simulink model "deadbeat_running_control"  (R2016b)
settings: configuration reference "Configuration1khz" (kept outside this file)
undefined symbols (not defined in the file or in its folder): A_kalman_no_position, A_kalman_transverse, A_kalman_vertical, A_lpf_accelerometer, A_lpf_contact, A_lpf_imu, A_lpf_lateral_angle, B1_lpf_accelerometer, B1_lpf_contact, B1_lpf_imu, B1_lpf_lateral_angle, B2_lpf_accelerometer, B2_lpf_contact, B2_lpf_imu, B2_lpf_lateral_angle, B_dx_versus_x0, B_kalman_no_position, B_kalman_transverse, B_kalman_vertical, backwards_K_sag_of_t, backwards_P_sag_of_t, C_kalman_no_position, C_kalman_transverse, C_kalman_vertical, com_leg_motor, com_torso, contact_threshold, d_ankle_to_foot, d_vertical_com, desired_com_forward_velocity, desired_com_lateral_velocity, desired_standing_torso_pitch, desired_standing_torso_roll, desired_standing_z, desired_torso_pitch, desired_torso_roll, DiscIntNeverNeededParam, Discrete, enable_bouncing, fdesignblkfcn, flight_duration, forward_dx_of_dxstar, forward_x_of_dxstar, g, gcbh, HIP_MTR_MAX_CONT_TORQUE, HIP_MTR_MAX_TORQUE, i_leg_motor, i_robot, i_torso, initial_dx_estimate, initial_dx_takeoff_history, initial_dx_touchdown_history, initial_dy_estimate, initial_dy_takeoff_history, initial_dy_touchdown_history, initial_dz_estimate, initial_leg_selection, initial_target_dx_history, initial_target_dy_history ... (+80)
libraries: simulink x22, ctrlSharedLib x4, dsparch4 x2
(part 1 of 7)
settings Model: Creator=wmartin  LastModifiedBy=Will
settings ConfigSetRef: SourceLocation=Base Workspace

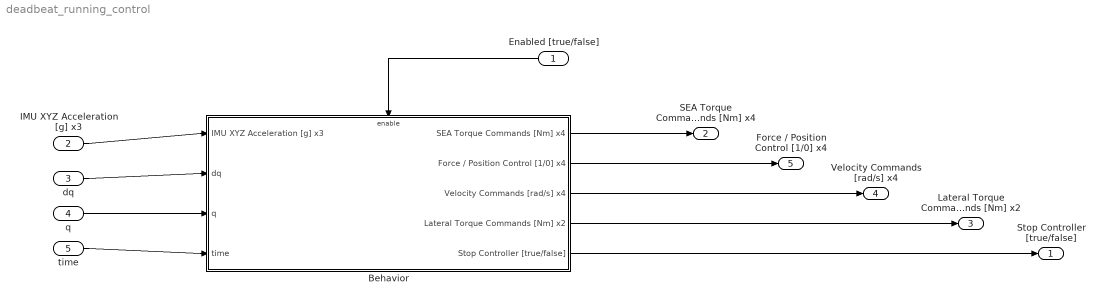
== system deadbeat_running_control ==
  Enabled [true/false] : Inport  OutDataTypeStr=boolean  PortDimensions=1  SampleTime=sample_time  Interpolate=off
  IMU XYZ Acceleration [g] x3 : Inport  Port=2  OutDataTypeStr=double  PortDimensions=3  SampleTime=[0.001,0]  Interpolate=off
  dq : Inport  Port=3  OutDataTypeStr=double  PortDimensions=13  SampleTime=[0.001,0]  Interpolate=off
  q : Inport  Port=4  OutDataTypeStr=double  PortDimensions=13  SampleTime=[0.001,0]  Interpolate=off
  time : Inport  Port=5  OutDataTypeStr=double  PortDimensions=1  SampleTime=sample_time  Interpolate=off
  Behavior : Subsystem
  Stop Controller [true/false] : Outport  OutDataTypeStr=boolean  PortDimensions=1  SampleTime=[0.001,0]  OutputWhenDisabled=reset  InitialOutput=[0 0 0 0 0 0]
  SEA Torque Commands [Nm] x4 : Outport  Port=2  OutDataTypeStr=double  PortDimensions=4  SampleTime=[0.001,0]  OutputWhenDisabled=reset  InitialOutput=[0 0 0 0 0 0]
  Lateral Torque Commands [Nm] x2 : Outport  Port=3  OutDataTypeStr=double  PortDimensions=2  SampleTime=[0.001,0]  OutputWhenDisabled=reset  InitialOutput=[0 0 0 0 0 0]
  Velocity Commands [rad/s] x4 : Outport  Port=4  OutDataTypeStr=double  PortDimensions=4  SampleTime=[0.001,0]  OutputWhenDisabled=reset  InitialOutput=[0 0 0 0 0 0]
  Force / Position Control [1/0] x4 : Outport  Port=5  OutDataTypeStr=boolean  PortDimensions=4  SampleTime=[0.001,0]  OutputWhenDisabled=reset  InitialOutput=[0 0 0 0 0 0]
  wires:
  IMU XYZ Acceleration [g] x3/1 -> Behavior/1(IMU XYZ Acceleration [g] x3)
  dq/1 -> Behavior/2(dq)
  q/1 -> Behavior/3(q)
  Behavior/1(SEA Torque Commands [Nm] x4) -> SEA Torque Commands [Nm] x4/1
  Behavior/2(Force / Position Control [1/0] x4) -> Force / Position Control [1/0] x4/1
  Behavior/3(Velocity Commands [rad/s] x4) -> Velocity Commands [rad/s] x4/1
  Behavior/4(Lateral Torque Commands [Nm] x2) -> Lateral Torque Commands [Nm] x2/1
  time/1 -> Behavior/4(time)
  Enabled [true/false]/1 -> Behavior/Enable
  Behavior/5(Stop Controller [true/false]) -> Stop Controller [true/false]/1

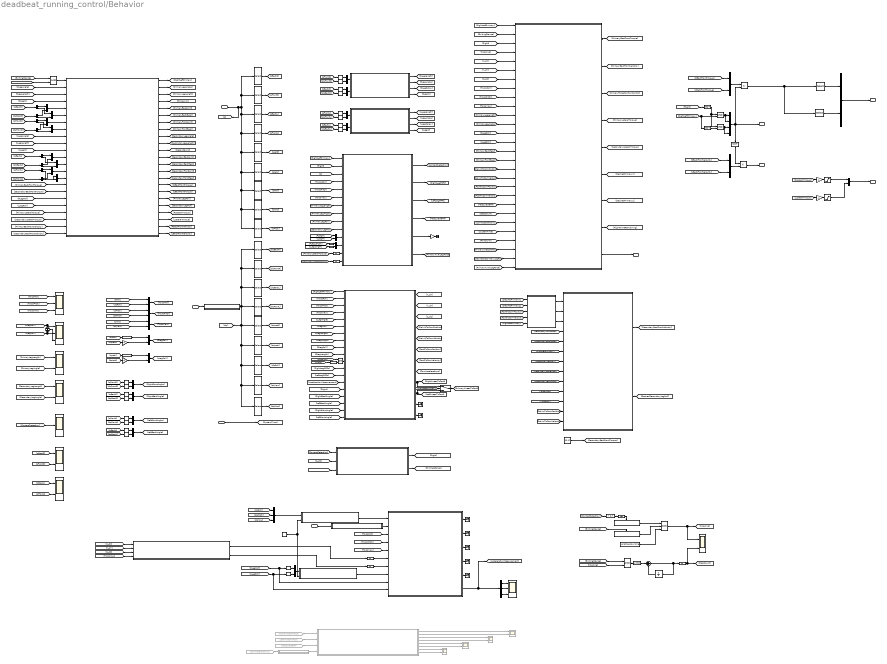
== system deadbeat_running_control/Behavior ==
  note: Signal Routing
  note: Begin Control
  note: Position & Velocity Estimation
  note: Force Estimation
  note: Leg/Spring Measurements
  note: Torque Commands
  note: Secondary Leg Behavior
  note: Primary Leg + Lateral Behavior
  note: Inputs
  note: q Order:
      |
      | backJointR
      | backGearR
      | frontJointR
      | frontGearR
      |
      | backJointL
      | backGearL
      | frontJointL
      | frontGearL
      |
      | latR
      | latL
      |
      | torsoRoll
      | torsoYaw
      | torsoPitch
  note: Angle Conversions
  note: Contact Estimation
  note: Logging
  note: Acceleration Measurement
  note: Knee Torque Estimation
  IMU XYZ Acceleration [g] x3 : Inport  OutDataTypeStr=double  PortDimensions=3  SampleTime=[0.001,0]
  dq : Inport  Port=2  OutDataTypeStr=double  PortDimensions=13  SampleTime=[0.001,0]
  q : Inport  Port=3  OutDataTypeStr=double  PortDimensions=13  SampleTime=[0.001,0]
  time : Inport  Port=4  OutDataTypeStr=double  PortDimensions=1  SampleTime=[0.001,0]
  Enable : EnablePort  PropagateVarSize=During execution  ShowOutputPort=on
  At Least One Stance Detected : Subsystem
  Atrias Swing control : Subsystem
  COM Acceleration Measurement : Scope  NumInputPorts=3
  Compare To Constant : simulink/Logic and Bit Operations/Compare To Constant  relop=>  const=0.7  OutDataTypeStr=boolean
  Compute Body Frame Accelerations : Subsystem
  Compute COM Translational Acceleration (IMU uses non-rotating measurement frame) : MATLAB Function  TreatAsAtomicUnit=on
  Compute Forces1 : Subsystem  Commented=on
  Compute World Frame COM Coordinates from Yawed Frame : MATLAB Function  TreatAsAtomicUnit=on
  Constant : Constant  Value=[0 0]
  Constant1 : Constant  Value=enable_bouncing
  Contact : Scope
  Contact State Machine : Subsystem
  Data Type Conversion : DataTypeConversion  OutDataTypeStr=uint32
  Demux : Demux  Outputs=3
  Demux{3..10} (8 alike) : Demux  Outputs=2
  Desired Secondary Swing Targets : Subsystem
  Estimate Angular Accelerations2 : Subsystem
  Estimate Angular Accelerations3 : Subsystem
  Exited Stance : Subsystem
  Filter Velocities : Subsystem
  Force Estimation : Subsystem
  From40 : From  Commented=on  GotoTag=RightKneesToFoot
  From56 : From  Commented=on  GotoTag=LeftKneesToFoot
  From57 : From  Commented=on  GotoTag=MeasuredGRF
  From76 : From  Commented=on  GotoTag=ComAccelerations
  Gain{1..2,12..13} (4 alike) : Gain  Gain=-1
  Hopping / Steps : Scope  NumInputPorts=2
  Knee Torques : MATLAB Function  Commented=on  TreatAsAtomicUnit=on
  L Knee Torques from Accelerometer : Scope  Commented=on  NumInputPorts=2
  L Knee Torques from Forward Dynamics : Scope  Commented=on  NumInputPorts=2
  L Leg Calculator : Subsystem
  Left Lateral Torque Saturation : Saturate  UpperLimit=max_torque_lateral  LowerLimit=-max_torque_lateral
      settings: AttributesFormatString=Top: %<UpperLimit>\nBottom: %<LowerLimit>
  Left Leg Fourbar Positions : Scope  NumInputPorts=2
  Logical Operator : Logic  IconShape=distinctive  AllPortsSameDT=off  OutDataTypeStr=boolean
  Logical Operator1 : Logic  AllPortsSameDT=off  OutDataTypeStr=boolean
  Logical Operator2 : Logic  Operator=OR  AllPortsSameDT=off  OutDataTypeStr=boolean
  Logical Operator3 : Logic  Inputs=3  AllPortsSameDT=off  OutDataTypeStr=boolean
  Logical Operator{4,6,8..9} (4 alike) : Logic  Operator=NOT  AllPortsSameDT=off  OutDataTypeStr=boolean
  Logical Operator5 : Logic  AllPortsSameDT=off  OutDataTypeStr=boolean
  Logical Operator7 : Logic  AllPortsSameDT=off  OutDataTypeStr=boolean
  Mux{,1..2,4..27,30} (28 alike) : Mux  Inputs=2
  Mux28 : Mux  Inputs=3
  Mux3 : Mux
  Primary Leg Length / Angle : Scope  NumInputPorts=2
  Primary Secondary Leg Swap : Subsystem
  Primary and Lateral Behavior : Subsystem
  Product : Product
  Product1 : Product
  R Knee Torques from Accelerometer : Scope  Commented=on  NumInputPorts=2
  R Knee Torques from Forward Dynamics : Scope  Commented=on  NumInputPorts=2
  R Leg Calculator : Subsystem
  Right Lateral Torque Saturation : Saturate  UpperLimit=max_torque_lateral  LowerLimit=-max_torque_lateral
      settings: AttributesFormatString=Top: %<UpperLimit>\nBottom: %<LowerLimit>
  Right Left Symmetry Leg Roll : Scope  NumInputPorts=3
  Right Leg Fourbar Positions : Scope  NumInputPorts=2
  Roll Pitch Yaw : Scope  NumInputPorts=3
  Secondary Leg Length / Angle : Scope  NumInputPorts=2
  Selector : Selector  InputPortWidth=4  IndexOptions=Index vector (dialog)  Indices=[1 2]  OutputSizes=1
  Selector1 : Selector  InputPortWidth=13  IndexOptions=Index vector (dialog)  Indices=[10]  OutputSizes=1
  Selector10 : Selector  InputPortWidth=13  IndexOptions=Index vector (dialog)  Indices=[7 8]  OutputSizes=1
  Selector11 : Selector  InputPortWidth=13  IndexOptions=Index vector (dialog)  Indices=[9]  OutputSizes=1
  Selector12 : Selector  InputPortWidth=13  IndexOptions=Index vector (dialog)  Indices=[1 2]  OutputSizes=1
  Selector13 : Selector  InputPortWidth=13  IndexOptions=Index vector (dialog)  Indices=[3 4]  OutputSizes=1
  Selector{14..17,19,24..27,29..37} (18 alike) : Selector  InputPortWidth=2  IndexOptions=Index vector (dialog)  Indices=[1]  OutputSizes=1
  Selector18 : Selector  InputPortWidth=13  IndexOptions=Index vector (dialog)  Indices=[13]  OutputSizes=1
  Selector2 : Selector  InputPortWidth=13  IndexOptions=Index vector (dialog)  Indices=[5 6]  OutputSizes=1
  Selector20 : Selector  InputPortWidth=13  IndexOptions=Index vector (dialog)  Indices=[13]  OutputSizes=1
  Selector21 : Selector  InputPortWidth=13  IndexOptions=Index vector (dialog)  Indices=[11]  OutputSizes=1
  Selector22 : Selector  InputPortWidth=13  IndexOptions=Index vector (dialog)  Indices=[12]  OutputSizes=1
  Selector23 : Selector  InputPortWidth=13  IndexOptions=Index vector (dialog)  Indices=[11]  OutputSizes=1
  Selector28 : Selector  InputPortWidth=13  IndexOptions=Index vector (dialog)  Indices=[12]  OutputSizes=1
  Selector3 : Selector  InputPortWidth=4  IndexOptions=Index vector (dialog)  Indices=[3 4]  OutputSizes=1
  Selector4 : Selector  InputPortWidth=13  IndexOptions=Index vector (dialog)  Indices=[7 8]  OutputSizes=1
  Selector41 : Selector  InputPortWidth=2  IndexOptions=Index vector (dialog)  Indices=[2]  OutputSizes=1
  Selector42 : Selector  InputPortWidth=2  IndexOptions=Index vector (dialog)  Indices=[2]  OutputSizes=1
  Selector5 : Selector  InputPortWidth=13  IndexOptions=Index vector (dialog)  Indices=[9]  OutputSizes=1
  Selector6 : Selector  InputPortWidth=13  IndexOptions=Index vector (dialog)  Indices=[1 2]  OutputSizes=1
  Selector7 : Selector  InputPortWidth=13  IndexOptions=Index vector (dialog)  Indices=[3 4]  OutputSizes=1
  Selector8 : Selector  InputPortWidth=13  IndexOptions=Index vector (dialog)  Indices=[10]  OutputSizes=1
  Selector9 : Selector  InputPortWidth=13  IndexOptions=Index vector (dialog)  Indices=[5 6]  OutputSizes=1
  State Estimation : Subsystem
  Sum1 : Sum  Inputs=|++  OutMin=0
  Sum3 : Sum  Inputs=-|+
  Switch : Switch  Criteria=u2 ~= 0
  Terminator{,1..7} (8 alike) : Terminator
  Unit Delay : UnitDelay  SampleTime=-1
  Unit Delay{1..6} (6 alike) : UnitDelay  SampleTime=sample_time
  lateral_coordinates : Fcn  Expr=pi/2-u
  lateral_coordinates1 : Fcn  Expr=pi/2-u
  torso_roll_acceleration : Gain
  SEA Torque Commands [Nm] x4 : Outport  OutDataTypeStr=double  PortDimensions=4  SampleTime=[0.001,0]  OutputWhenDisabled=reset  InitialOutput=[0 0 0 0]
  Force / Position Control [1/0] x4 : Outport  Port=2  OutDataTypeStr=boolean  PortDimensions=4  SampleTime=[0.001,0]  OutputWhenDisabled=reset  InitialOutput=[0 0 0 0]
  Velocity Commands [rad/s] x4 : Outport  Port=3  OutDataTypeStr=double  PortDimensions=4  SampleTime=[0.001,0]  OutputWhenDisabled=reset  InitialOutput=[0 0 0 0]
  Lateral Torque Commands [Nm] x2 : Outport  Port=4  OutDataTypeStr=double  PortDimensions=2  SampleTime=[0.001,0]  OutputWhenDisabled=reset  InitialOutput=[0 0]
  Stop Controller [true/false] : Outport  Port=5  OutDataTypeStr=boolean  PortDimensions=1  SampleTime=[0.001,0]  OutputWhenDisabled=reset  InitialOutput=0
  wires:
  [SecondaryLateralTorque] -> Unit Delay4/1
  Unit Delay3/1 -> Force Estimation/13(Primary Lateral Torque [Nm])
  Gain1/1 -> Left Lateral Torque Saturation/1
  [RLegLength] -> Selector19/1
  [RLegW] -> Mux19/1
  [PrimaryLateralTorque] -> Unit Delay3/1
  [PrimaryLateralTorque] -> Primary Secondary Leg Swap/20(Primary Lateral Torque [Nm])
  [SecondaryLegRoll] -> Force Estimation/10(Secondary Leg Roll [rad rad/s])
  Mux20/1 -> Force Estimation/12(Leg Length Right/Left [m m])
  Gain2/1 -> Right Lateral Torque Saturation/1
  [LLegRoll] -> Primary and Lateral Behavior/14(Left Leg Roll [rad rad/s])
  Selector29/1 -> Mux20/2
  Primary Secondary Leg Swap/20(Right Lateral Torque [Nm]) -> [RLateralTorque]
  Force Estimation/5(Torso Roll Acceleration [rad/s^2]) -> torso_roll_acceleration/1
  Primary and Lateral Behavior/4(Primary Lateral Torque [Nm]) -> [PrimaryLateralTorque]
  [SecondaryLateralTorque] -> Primary Secondary Leg Swap/21(Secondary Lateral Torque [Nm])
  Mux19/1 -> Force Estimation/11(Leg Width Right/Left [m m])
  Primary Secondary Leg Swap/21(Left Lateral Torque [Nm]) -> [LLateralTorque]
  torso_roll_acceleration/1 -> Terminator6/1
  Unit Delay4/1 -> Force Estimation/14(Secondary Lateral Torque [Nm])
  [Y_dY] -> Primary and Lateral Behavior/6("[y,  dy] [m, m/s]")
  [LLegLength] -> Selector29/1
  [StepCount] -> Primary and Lateral Behavior/22(Steps Taken)
  Logical Operator3/1 -> [hopping], Hopping / Steps/1
  [TorsoYaw] -> Primary and Lateral Behavior/10(Torso Yaw [rad rad/s])
  [RLegRoll] -> Primary and Lateral Behavior/13(Right Leg Roll [rad rad/s])
  [MeasuredGRF] -> Primary and Lateral Behavior/21(Measured GRF [N N N])
  [TorsoRoll] -> Primary and Lateral Behavior/8(Torso Roll [rad rad/s])
  [Z_dZ] -> Primary and Lateral Behavior/7("[z, dz] [m, m/s]")
  Selector19/1 -> Mux20/1
  Primary and Lateral Behavior/5(Secondary Lateral Torque [Nm]) -> [SecondaryLateralTorque]
  [LLegW] -> Mux19/2
  [RLegRoll] -> Right Left Symmetry Leg Roll/1, Sum3/1
  Mux23/1 -> [TorsoRoll]
  Mux7/1 -> [TorsoPitch]
  Contact State Machine/2(Exiting Stance [1/0]) -> [ExitingStance]
  [ContactDetection] -> Contact State Machine/1(Contact Factor [body weight])
  [PrimaryLegAngle] -> Primary and Lateral Behavior/12(Leg Angle [rad rad/s])
  [Z_dZ] -> Contact State Machine/2("[Z dZ] [m m/s]")
  [FootToComPosition] -> Primary and Lateral Behavior/19(Foot to COM Position [m m m])
  [PrimaryLegLength] -> Primary and Lateral Behavior/11(Leg Length [m m/s])
  [PrimaryFrontGear] -> Primary and Lateral Behavior/16(Primary Front Gear [rad rad/s])
  [hopping] -> Primary and Lateral Behavior/4(Hopping [1/0])
  [FootToComVelocity] -> Primary and Lateral Behavior/20(Foot to COM Velocity [m m m])
  [TorsoPitch] -> Roll Pitch Yaw/2
  [LLegRoll] -> Right Left Symmetry Leg Roll/2, Sum3/2
  [flight] -> Primary and Lateral Behavior/3(Flight [1/0])
  [TorsoPitch] -> Primary and Lateral Behavior/9(Torso Pitch [rad rad/s])
  Sum3/1 -> Right Left Symmetry Leg Roll/3
  [PrimaryLegLength] -> Primary Leg Length / Angle/1
  [PelvisToComPosition] -> Primary and Lateral Behavior/17(Pelvis to COM Position [m m m])
  [PrimaryLegAngle] -> Primary Leg Length / Angle/2
  [SecondaryLegLength] -> Secondary Leg Length / Angle/1
  [SecondaryLegAngle] -> Secondary Leg Length / Angle/2
  [ContactDetection] -> Contact/1
  Contact State Machine/1(flight [1/0]) -> [flight]
  [RightLeftPrimary] -> Primary and Lateral Behavior/1(Right/Left [1/0])
  [X_dX] -> Primary and Lateral Behavior/5("[x, dx] [m, m/s]")
  [ExitingStance] -> Primary and Lateral Behavior/2(Exiting Stance [1/0])
  [TorsoRoll] -> Roll Pitch Yaw/1
  Mux21/1 -> [TorsoYaw]
  [PelvisToComVelocity] -> Primary and Lateral Behavior/18(Pelvis to COM Velocity [m m m])
  [PrimaryBackGear] -> Primary and Lateral Behavior/15(Primary Back Gear [rad rad/s])
  [TorsoYaw] -> Roll Pitch Yaw/3
  [dqLatL] -> Gain13/1
  Selector21/1 -> [dqRoll]
  Selector9/1 -> [dqBackL]
  [qYaw] -> Mux21/1
  time/1 -> [SystemTime]
  [dqLatR] -> Gain12/1
  lateral_coordinates/1 -> Mux22/1
  [ComAccelerations] -> Primary and Lateral Behavior/23(COM XYZ Acceleration [m/s^2] x3)
  [qBackL] -> Left Leg Fourbar Positions/1
  Gain12/1 -> Mux22/2
  [dqPitch] -> Mux7/2
  Selector20/1 -> [dqPitch]
  [qRoll] -> Mux23/1
  [qPitch] -> Mux7/1
  lateral_coordinates1/1 -> Mux24/1
  Selector10/1 -> [dqFrontL]
  [qBackR] -> Right Leg Fourbar Positions/1
  [qLatL] -> lateral_coordinates1/1
  Mux22/1 -> [RLegRoll]
  Gain13/1 -> Mux24/2
  Selector13/1 -> [dqFrontR]
  Selector11/1 -> [dqLatR]
  Mux24/1 -> [LLegRoll]
  [dqRoll] -> Mux23/2
  Selector8/1 -> [dqLatL]
  [dqYaw] -> Mux21/2
  [qLatR] -> lateral_coordinates/1
  [qFrontR] -> Right Leg Fourbar Positions/2
  Selector12/1 -> [dqBackR]
  Selector22/1 -> [dqYaw]
  [qFrontL] -> Left Leg Fourbar Positions/2
  Atrias Swing control/2(Desired Swing Beta [rad rad/s rad/s^2]) -> [DesiredSecondaryLegRoll]
  [DesiredPrimaryX] -> Desired Secondary Swing Targets/1(Desired Primary X)
  Atrias Swing control/1(Secondary Back/Front Motor Velocity [rad/s rad/s]) -> [SecondaryBackFrontVelocity]
  Desired Secondary Swing Targets/2(Desired Y) -> Atrias Swing control/2(Y Desired [m m/s m/s^2])
  State Estimation/12(Foot to COM Velocity Global [m/s m/s m/s]) -> Terminator1/1
  Primary and Lateral Behavior/6("Desired Primary X [m, m/s, m/s^2]") -> [DesiredPrimaryX]
  Desired Secondary Swing Targets/3(Desired Z) -> Atrias Swing control/3(Z Desired [m m/s m/s^2])
  Desired Secondary Swing Targets/1(Desired X) -> Atrias Swing control/1(X Desired [m m/s m/s^2])
  Primary and Lateral Behavior/7("Desired Primary Z [m, m/s, m/s^2]") -> [DesiredPrimaryZ]
  State Estimation/11(Foot to COM Position Global [m m m]) -> Terminator/1
  [DesiredPrimaryZ] -> Desired Secondary Swing Targets/2(Desired Primary Z)
  [FootToComPosition] -> Desired Secondary Swing Targets/3(Primary X,Y,Z)
  [PrimaryAxialLegForce] -> Primary and Lateral Behavior/28(Primary Axial Leg Force [N])
  Force Estimation/6(Primary Axial Leg Force) -> [PrimaryAxialLegForce]
  [FootToComVelocity] -> Desired Secondary Swing Targets/4(Primary dX,dY,dZ)
  [DesiredSecondaryLegRoll] -> Primary and Lateral Behavior/27(Desired Secondary Leg Roll [rad rad/s rad/s^2])
  [RightLeftPrimary] -> Desired Secondary Swing Targets/5(Right / Left)
  [PelvisToComVelocity] -> Atrias Swing control/13(Pelvis to COM Velocity [m/s m/s m/s])
  [PelvisToComPosition] -> Atrias Swing control/12(Pelvis to COM Position [m m m])
  Compute World Frame COM Coordinates from Yawed Frame/2(com_velocity_world) -> Unit Delay6/1
  Selector42/1 -> Mux30/2
  [LLegRoll] -> Selector42/1, Compute COM Translational Acceleration (IMU uses non-rotating measurement frame)/10(left_hip_roll)
  [TorsoYaw] -> Compute COM Translational Acceleration (IMU uses non-rotating measurement frame)/5(torso_yaw)
  [TorsoRoll] -> Atrias Swing control/11(Torso Roll [rad rad/s])
  [SecondaryLegLength] -> Atrias Swing control/8(Secondary Leg Length [m m/s])
  [SecondaryLegAngle] -> Atrias Swing control/9(Secondary Leg Angle [rad rad/s])
  Compute World Frame COM Coordinates from Yawed Frame/1(com_position_world) -> Unit Delay5/1
  Unit Delay6/1 -> Compute COM Translational Acceleration (IMU uses non-rotating measurement frame)/7(com_velocity_world)
  Unit Delay5/1 -> Compute COM Translational Acceleration (IMU uses non-rotating measurement frame)/6(com_position_world)
  [TorsoPitch] -> Atrias Swing control/10(Torso Pitch [rad rad/s])
  [RightLeftPrimary] -> Atrias Swing control/6(Right or Left Stance [1 or 0])
  [TorsoYaw] -> Compute World Frame COM Coordinates from Yawed Frame/4(torso_yaw)
  [X_dX] -> Compute World Frame COM Coordinates from Yawed Frame/1(X_dX)
  Estimate Angular Accelerations3/1(Angular Accelerations [rad/s^2] x2) -> Compute COM Translational Acceleration (IMU uses non-rotating measurement frame)/8(hip_roll_accelerations)
  Mux30/1 -> Estimate Angular Accelerations3/1(Angular Velocities [rad/s] x2)
  [SecondaryLegRoll] -> Atrias Swing control/7(Secondary Leg Roll [rad rad/s])
  [Y_dY] -> Compute World Frame COM Coordinates from Yawed Frame/2(Y_dY)
  Selector41/1 -> Mux30/1
  Estimate Angular Accelerations2/1(Angular Accelerations [rad/s^2] x3) -> Compute COM Translational Acceleration (IMU uses non-rotating measurement frame)/1(torso_angular_accelerations)
  IMU XYZ Acceleration [g] x3/1 -> Compute Body Frame Accelerations/1(accelerometer [g] x3)
  [RLegRoll] -> Selector41/1, Compute COM Translational Acceleration (IMU uses non-rotating measurement frame)/9(right_hip_roll)
  Mux28/1 -> Estimate Angular Accelerations2/1(Angular Velocities [rad/s] x3)
  [dqYaw] -> Mux28/3
  [Z_dZ] -> Compute World Frame COM Coordinates from Yawed Frame/3(Z_dZ)
  Enable/1 -> Estimate Angular Accelerations2/2(Enabled), Estimate Angular Accelerations3/2(Enabled)
  [SecondaryBackGear] -> Atrias Swing control/5(Secondary Back Gear [rad rad/s])
  [dqPitch] -> Mux28/2
  [dqRoll] -> Mux28/1
  [SecondaryFrontGear] -> Atrias Swing control/4(Secondary Front Gear [rad rad/s])
  Compute COM Translational Acceleration (IMU uses non-rotating measurement frame)/6(com_acceleration_yawed) -> Demux/1, [AccelerationMeasurement]
  Logical Operator2/1 -> State Estimation/11(Enable Kalman Filtering [1/0])
  [RightLegGRFs] -> State Estimation/12(Right GRF [X Y Z] [N N N])
  [RLegAngle] -> State Estimation/8(Right Leg Sagittal Angle [rad rad/s])
  Switch/1 -> [PrimaryKneesToFoot]
  State Estimation/8(COM Acceleration [m/s^2] x3) -> [ComAccelerations]
  State Estimation/1("Horizontal COM [m, m/s]") -> [X_dX]
  [RLegRoll] -> State Estimation/9(Right Leg Roll [rad rad/s])
  [AccelerationMeasurement] -> State Estimation/14(" Acceleration Measurement [m/s^2] x3")
  [LeftFrontAngle] -> State Estimation/19(Left Front [rad rad/s])
  [RightBackAngle] -> State Estimation/16(Right Back [rad rad/s])
  Demux/3 -> COM Acceleration Measurement/3
  [RightLeftPrimary] -> Switch/2
  [TorsoRoll] -> Compute COM Translational Acceleration (IMU uses non-rotating measurement frame)/3(torso_roll)
  [RLegLength] -> State Estimation/10(Right Leg Length [m m/s])
  [RightFrontAngle] -> State Estimation/18(Right Front [rad rad/s])
  [TorsoPitch] -> Compute COM Translational Acceleration (IMU uses non-rotating measurement frame)/4(torso_pitch)
  Demux/2 -> COM Acceleration Measurement/2
  [TorsoRoll] -> State Estimation/2(Torso Roll [rad rad/s])
  [TorsoPitch] -> State Estimation/3(Torso Pitch [rad rad/s])
  Demux/1 -> COM Acceleration Measurement/1
  [LLegRoll] -> State Estimation/6(Left Leg Roll [rad rad/s])
  [LLegLength] -> State Estimation/7(Left Leg Length [m m/s])
  [LLegAngle] -> State Estimation/5(Left Leg Sagittal Angle [rad rad/s])
  [RightLeftPrimary] -> State Estimation/1(Right or Left [1/0])
  State Estimation/9(Right Knees to Foot [m m m] x2) -> [RightKneesToFoot], Switch/1
  State Estimation/10(Left Knees to Foot [m m m] x2) -> Switch/3, [LeftKneesToFoot]
  [LeftBackAngle] -> State Estimation/17(Left Back [rad rad/s])
  State Estimation/3("Vertical COM [m, m/s]") -> [Z_dZ]
  Primary and Lateral Behavior/3(Primary Force or Position Control [1/0]) -> [PrimaryForcePositionControl]
  Logical Operator/1 -> Primary Secondary Leg Swap/1(Exiting Stance [1/0])
  [flight] -> Logical Operator4/1
  Primary and Lateral Behavior/1(Primary Back/Front SEA Torques [Nm] x2) -> [PrimaryBackFrontTorque]
  Sum1/1 -> Unit Delay2/1, Unit Delay/1
  Primary Secondary Leg Swap/16(R Back/Front SEA Torque [Nm Nm]) -> [RBackFrontTorque]
  State Estimation/4(Pelvis to COM Position [m m m]) -> [PelvisToComPosition]
  Logical Operator1/1 -> Data Type Conversion/1
  Primary Secondary Leg Swap/13(Secondary Back Gear [rad rad/s]) -> [SecondaryBackGear]
  [TorsoYaw] -> State Estimation/4(Torso Yaw [rad rad/s])
  [hopping] -> Logical Operator2/1
  [ExitingStance] -> Exited Stance/Enable
  [LeftLegGRFs] -> State Estimation/13(Left GRF [X Y Z] [N N N])
  State Estimation/5(Pelvis to COM Velocity [m/s m/s m/s]) -> [PelvisToComVelocity]
  [flight] -> State Estimation/15(Flight [1/0])
  State Estimation/7(Foot to COM Velocity [m/s m/s m/s]) -> [FootToComVelocity]
  Unit Delay/1 -> Sum1/2
  [RLateralTorque] -> Gain2/1
  Primary Secondary Leg Swap/17(L Back/Front SEA Torque [Nm Nm]) -> [LBackFrontTorque]
  State Estimation/2("Lateral COM [m, m/s]") -> [Y_dY]
  Logical Operator4/1 -> Logical Operator2/2
  Primary Secondary Leg Swap/11(Secondary Leg w [m]) -> [SecondaryW]
  Primary Secondary Leg Swap/15(Secondary Front Gear [rad rad/s]) -> [SecondaryFrontGear]
  State Estimation/6(Foot to COM Position [m m m]) -> [FootToComPosition]
  Primary Secondary Leg Swap/14(Secondary Front Joint [rad rad/s]) -> [SecondaryFrontJoint]
  Primary Secondary Leg Swap/1(Right/Left Primary [1/0]) -> [RightLeftPrimary]
  Data Type Conversion/1 -> Sum1/1
  Primary Secondary Leg Swap/12(Secondary Back Joint [rad rad/s]) -> [SecondaryBackJoint]
  Primary Secondary Leg Swap/8(Primary Front Gear [rad rad/s]) -> [PrimaryFrontGear]
  Primary Secondary Leg Swap/7(Primary Front Joint [rad rad/s]) -> [PrimaryFrontJoint]
  Primary Secondary Leg Swap/6(Primary Back Gear [rad rad/s]) -> [PrimaryBackGear]
  Mux15/1 -> Primary Secondary Leg Swap/15(L Front Gear [rad rad/s])
  Mux12/1 -> Primary Secondary Leg Swap/8(R Front Gear [rad rad/s])
  Mux11/1 -> Primary Secondary Leg Swap/7(R Front Joint [rad rad/s])
  Demux7/1 -> Mux14/1
  Mux10/1 -> Primary Secondary Leg Swap/6(R Back Gear [rad rad/s])
  Demux7/2 -> Mux15/1
  [SecondaryBackFrontTorque] -> Primary Secondary Leg Swap/17(Secondary Back/Front SEA Torque [Nm Nm])
  Mux14/1 -> Primary Secondary Leg Swap/14(L Front Joint [rad rad/s])
  Primary Secondary Leg Swap/5(Primary Back Joint [rad rad/s]) -> [PrimaryBackJoint]
  Demux10/2 -> Mux13/1
  Mux16/1 -> Primary Secondary Leg Swap/12(L Back Joint [rad rad/s])
  Demux6/2 -> Mux10/1
  Demux5/1 -> Mux9/2
  [qBackR] -> Demux6/1
  [dqBackL] -> Demux9/1
  [qBackL] -> Demux10/1
  Mux13/1 -> Primary Secondary Leg Swap/13(L Back Gear [rad rad/s])
  [dqFrontL] -> Demux8/1
  Demux8/2 -> Mux15/2
  Demux8/1 -> Mux14/2
  [dqBackR] -> Demux5/1
  Demux4/2 -> Mux12/2
  [qFrontL] -> Demux7/1
  Demux4/1 -> Mux11/2
  Demux10/1 -> Mux16/1
  Demux9/2 -> Mux13/2
  [PrimaryBackFrontTorque] -> Primary Secondary Leg Swap/16(Primary Back/Front SEA Torque [Nm Nm])
  Demux6/1 -> Mux9/1
  Demux5/2 -> Mux10/2
  Demux9/1 -> Mux16/2
  Demux3/2 -> Mux12/1
  Demux3/1 -> Mux11/1
  Selector27/1 -> Mux4/2
  Selector23/1 -> [qRoll]
  Mux9/1 -> Primary Secondary Leg Swap/5(R Back Joint [rad rad/s])
  [LLegLength] -> Primary Secondary Leg Swap/10(L Leg Length [m m/s])
  [dqFrontR] -> Demux4/1
  [qFrontR] -> Demux3/1
  [qBackL] -> Selector26/1
  Primary Secondary Leg Swap/2(Primary Leg Angle [rad rad/s]) -> [PrimaryLegAngle]
  [RLegLength] -> Primary Secondary Leg Swap/3(R Leg Length [m m/s])
  Selector25/1 -> Mux5/2
  Mux4/1 -> L Leg Calculator/2(Back [rad rad/s])
  [dqBackL] -> Selector27/1
  L Leg Calculator/4(w [m]) -> [LLegW]
  Mux5/1 -> L Leg Calculator/1(Front [rad rad/s])
  q/1 -> Selector6/1, Selector7/1, Selector2/1, Selector4/1, Selector5/1, Selector18/1, Selector28/1, Selector23/1, Selector1/1, [q]
  Selector24/1 -> Mux5/1
  [LLegAngle] -> Primary Secondary Leg Swap/9(L Leg Angle [rad rad/s])
  [LLegW] -> Primary Secondary Leg Swap/11(L Leg w [m])
  Primary Secondary Leg Swap/3(Primary Leg Length [m m/s]) -> [PrimaryLegLength]
  Primary Secondary Leg Swap/4(Primary Leg w [m]) -> [PrimaryW]
  Primary Secondary Leg Swap/10(Secondary Leg Length [rad rad/s]) -> [SecondaryLegLength]
  R Leg Calculator/4(w [m]) -> [RLegW]
  Selector26/1 -> Mux4/1
  L Leg Calculator/3(Leg Splay [rad rad/s]) -> [LLegSplay]
  L Leg Calculator/2(Leg Angle [rad rad/s]) -> [LLegAngle]
  L Leg Calculator/1("Leg Length [m m/s] ") -> [LLegLength]
  [qFrontL] -> Selector24/1
  Selector18/1 -> [qPitch]
  [dqFrontL] -> Selector25/1
  Primary Secondary Leg Swap/9(Secondary Leg Angle [rad rad/s]) -> [SecondaryLegAngle]
  [RLegW] -> Primary Secondary Leg Swap/4(R Leg w [m])
  [RLegAngle] -> Primary Secondary Leg Swap/2(R Leg Angle [rad rad/s])
  R Leg Calculator/3(Leg Splay [rad rad/s]) -> [RLegSplay]
  [dqBackR] -> Selector17/1
  Force Estimation/3(Left GRF [X Y Z] [N N N]) -> [LeftLegGRFs]
  Selector16/1 -> Mux1/1
  [LLateralTorque] -> Gain1/1
  Primary Secondary Leg Swap/19("Secondary Leg Roll [rad, rad/s]") -> [SecondaryLegRoll]
  Mux1/1 -> R Leg Calculator/2(Back [rad rad/s])
  Selector14/1 -> Mux2/1
  [qBackR] -> Selector16/1
  Selector2/1 -> [qBackL]
  Mux2/1 -> R Leg Calculator/1(Front [rad rad/s])
  Force Estimation/2(Right GRF [X Y Z] [N N N]) -> [RightLegGRFs]
  Selector4/1 -> [qFrontL]
  Selector5/1 -> [qLatR]
  Selector7/1 -> [qFrontR]
  Selector17/1 -> Mux1/2
  R Leg Calculator/2(Leg Angle [rad rad/s]) -> [RLegAngle]
  R Leg Calculator/1("Leg Length [m m/s] ") -> [RLegLength]
  Selector1/1 -> [qLatL]
  [dqFrontR] -> Selector15/1
  Selector6/1 -> [qBackR]
  [qFrontR] -> Selector14/1
  Force Estimation/1(Leg Plane Force for Contact Detection [body weight]) -> [ContactDetection]
  Force Estimation/4(GRF XYZ estimates [N N N]) -> [MeasuredGRF]
  [RLegRoll] -> Primary Secondary Leg Swap/18("Right Leg Roll [rad, rad/s]")
  Primary Secondary Leg Swap/18("Primary Leg Roll [rad, rad/s]") -> [PrimaryLegRoll]
  [LLegRoll] -> Primary Secondary Leg Swap/19("Left Leg Roll [rad, rad/s]")
  Unit Delay2/1 -> [StepCount], Hopping / Steps/2
  Selector28/1 -> [qYaw]
  Selector15/1 -> Mux2/2
  [PrimaryLegLength] -> Force Estimation/7(Primary Leg Length [m m/s])
  [PrimaryLegAngle] -> Force Estimation/8(Primary Leg Angle [rad rad/s])
  [PrimaryLegRoll] -> Force Estimation/9(Primary Leg Roll [rad rad/s])
  [ExitingStance] -> Logical Operator1/1
  [ExitingStance] -> Logical Operator/1
  [RightLeftPrimary] -> Force Estimation/1(Right/Left Primary)
  [flight] -> Force Estimation/2(Flight [1/0])
  [hopping] -> Logical Operator1/2
  [TorsoRoll] -> Force Estimation/4(Torso Roll [rad rad/s])
  [hopping] -> Logical Operator/2
  [TorsoYaw] -> Force Estimation/6(Torso Yaw [rad rad/s])
  [TorsoPitch] -> Force Estimation/5(Torso Pitch [rad rad/s])
  [q] -> Force Estimation/3(q)
  [RightLeftPrimary] -> Logical Operator5/2, Logical Operator8/1
  [RBackFrontVelocity] -> Mux6/1
  Unit Delay1/1 -> At Least One Stance Detected/Enable
  [LBackFrontVelocity] -> Mux6/2
  At Least One Stance Detected/1(Stance?) -> Logical Operator3/1
  [PrimaryBackFrontVelocity] -> Primary Secondary Leg Swap/22(Primary Front/Back Velocity [rad/s rad/s])
  [SecondaryBackFrontVelocity] -> Primary Secondary Leg Swap/23(Secondary Front/Back Velocity [rad/s rad/s])
  Primary Secondary Leg Swap/23(Left Front/Back Velocity [rad/s rad/s]) -> [LBackFrontVelocity]
  Selector3/1 -> Mux/2
  [SystemTime] -> Primary and Lateral Behavior/24(System Time [s])
  [PrimaryW] -> Primary and Lateral Behavior/25(Primary Leg Width [m])
  Exited Stance/1(Takeoff?) -> Logical Operator3/2
  [flight] -> Logical Operator6/1
  Compare To Constant/1 -> Unit Delay1/1
  Logical Operator8/1 -> Logical Operator7/2
  Logical Operator9/1 -> Product/1
  Mux/1 -> SEA Torque Commands [Nm] x4/1
  Product/1 -> Velocity Commands [rad/s] x4/1
  Primary and Lateral Behavior/2(Primary Back/Front Gear Velocities [rad/s] x2) -> [PrimaryBackFrontVelocity]
  [RBackFrontTorque] -> Mux8/1
  Mux6/1 -> Product/2
  [LBackFrontTorque] -> Mux8/2
  Product1/1 -> Selector/1, Selector3/1
  Primary Secondary Leg Swap/22(Right Front/Back Velocity [rad/s rad/s]) -> [RBackFrontVelocity]
  Selector/1 -> Mux/1
  Mux8/1 -> Product1/1
  Logical Operator7/1 -> Mux3/3, Mux3/4
  Constant/1 -> [SecondaryBackFrontTorque]
  Logical Operator5/1 -> Mux3/1, Mux3/2
  Logical Operator6/1 -> Logical Operator5/1, Logical Operator7/1
  Mux3/1 -> Force / Position Control [1/0] x4/1, Product1/2, Logical Operator9/1
  [ContactDetection] -> Compare To Constant/1
  [qFrontL] -> Selector34/1
  Knee Torques/6(left_back_knee_torques_from_fd) -> L Knee Torques from Forward Dynamics/2
  [dqFrontL] -> Selector35/1
  Selector34/1 -> Mux27/1
  Selector35/1 -> Mux27/2
  Knee Torques/2(right_back_knee_torques_from_fd) -> R Knee Torques from Forward Dynamics/2
  Compute Forces1/1(XYZ Force) -> Knee Torques/4(grf_from_accelerometer)
  From76/1 -> Compute Forces1/1(XYZ Acceleration)
  From40/1 -> Knee Torques/1(right_knees_to_foot)
  Knee Torques/1(right_front_knee_torques_from_fd) -> R Knee Torques from Forward Dynamics/1
  From57/1 -> Knee Torques/3(grf_from_seas)
  [dqBackR] -> Selector33/1
  [dqFrontR] -> Selector31/1
  Selector32/1 -> Mux17/1
  [qBackR] -> Selector32/1
  [dqBackL] -> Selector37/1
  Selector37/1 -> Mux26/2
  Selector31/1 -> Mux18/2
  [qBackL] -> Selector36/1
  Knee Torques/8(left_back_knee_torques_from_accelerometer) -> L Knee Torques from Accelerometer/2
  Selector36/1 -> Mux26/1
  [qFrontR] -> Selector30/1
  Knee Torques/4(right_back_knee_torques_from_accelerometer) -> R Knee Torques from Accelerometer/2
  Knee Torques/3(right_front_knee_torques_from_accelerometer) -> R Knee Torques from Accelerometer/1
  Selector30/1 -> Mux18/1
  Knee Torques/5(left_front_knee_torques_from_fd) -> L Knee Torques from Forward Dynamics/1
  Selector33/1 -> Mux17/2
  Knee Torques/7(left_front_knee_torques_from_accelerometer) -> L Knee Torques from Accelerometer/1
  From56/1 -> Knee Torques/2(left_knees_to_foot)
  [FlightTimeRemaining] -> Contact State Machine/3(Flight Time Remaining [s])
  Right Lateral Torque Saturation/1 -> Mux25/1
  Mux26/1 -> [LeftBackAngle]
  Mux17/1 -> [RightBackAngle]
  Mux18/1 -> [RightFrontAngle]
  dq/1 -> Filter Velocities/1(raw dq)
  Mux25/1 -> Lateral Torque Commands [Nm] x2/1
  [PrimaryKneesToFoot] -> Primary and Lateral Behavior/26(Primary Knees to Foot [m] x6)
  Mux27/1 -> [LeftFrontAngle]
  Compute Body Frame Accelerations/1(accelerations [m/s^2] x3) -> Compute COM Translational Acceleration (IMU uses non-rotating measurement frame)/2(imu_translational_accelerations_body)
  Filter Velocities/1(filtered dq) -> Selector9/1, Selector13/1, Selector12/1, Selector8/1, Selector22/1, Selector20/1, Selector21/1, Selector11/1, [dq], Selector10/1
  Left Lateral Torque Saturation/1 -> Mux25/2
  Compute COM Translational Acceleration (IMU uses non-rotating measurement frame)/2(torso_com_acceleration_world) -> Terminator3/1
  Compute COM Translational Acceleration (IMU uses non-rotating measurement frame)/3(pelvis_acceleration_world) -> Terminator4/1
  Compute COM Translational Acceleration (IMU uses non-rotating measurement frame)/4(right_hip_acceleration_world) -> Terminator5/1
  Compute COM Translational Acceleration (IMU uses non-rotating measurement frame)/1(com_acceleration_world) -> Terminator2/1
  Compute COM Translational Acceleration (IMU uses non-rotating measurement frame)/5(left_hip_acceleration_world) -> Terminator7/1
  Constant1/1 -> Logical Operator3/3
  Primary and Lateral Behavior/8(Flight Time Remaining [s]) -> [FlightTimeRemaining]
  Primary and Lateral Behavior/9(Stop Controller [true/false]) -> Stop Controller [true/false]/1

== system deadbeat_running_control/Behavior/At Least One Stance Detected ==
  Enable : EnablePort  StatesWhenEnabling=reset
  Constant : Constant
  Stance? : Outport  InitialOutput=[0]
  wires:
  Constant/1 -> Stance?/1

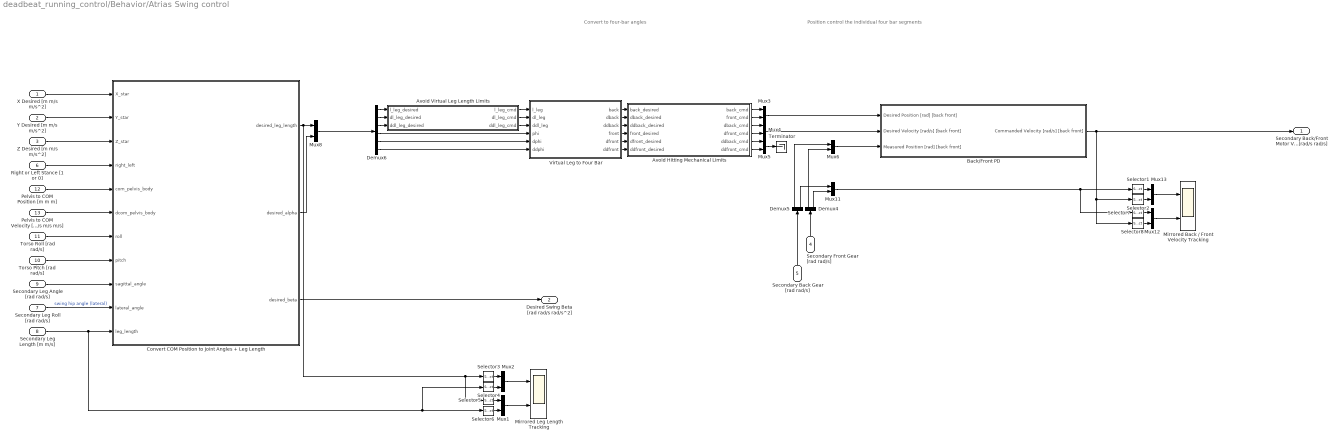
== system deadbeat_running_control/Behavior/Atrias Swing control ==
  note: Position control the
      | individual four bar segments
  note: Convert to
      | four-bar angles
  X Desired [m m/s m/s^2] : Inport
  Y Desired [m m/s m/s^2] : Inport  Port=2
  Z Desired [m m/s m/s^2] : Inport  Port=3
  Secondary Front Gear [rad rad/s] : Inport  Port=4
  Secondary Back Gear [rad rad/s] : Inport  Port=5
  Right or Left Stance [1 or 0] : Inport  Port=6
  Secondary Leg Roll [rad rad/s] : Inport  Port=7
  Secondary Leg Length [m m/s] : Inport  Port=8
  Secondary Leg Angle [rad rad/s] : Inport  Port=9
  Torso Pitch [rad rad/s] : Inport  Port=10
  Torso Roll [rad rad/s] : Inport  Port=11
  Pelvis to COM Position [m m m] : Inport  Port=12
  Pelvis to COM Velocity [m/s m/s m/s] : Inport  Port=13
  Avoid Hitting Mechanical Limits : MATLAB Function  TreatAsAtomicUnit=on
  Avoid Virtual Leg Length Limits : MATLAB Function  TreatAsAtomicUnit=on
  Back/Front PD : Subsystem
  "Convert COM Position to Joint Angles + Leg Length " : MATLAB Function  TreatAsAtomicUnit=on
  Demux4 : Demux  Outputs=2
  Demux5 : Demux  Outputs=2
  Demux6 : Demux  Outputs=6
  Mirrored Back / Front Velocity Tracking : Scope  NumInputPorts=2
  Mirrored Leg Length Tracking : Scope  NumInputPorts=2
  Mux{1..6,8,11..13} (10 alike) : Mux  Inputs=2
  Selector1 : Selector  InputPortWidth=2  IndexOptions=Index vector (dialog)  Indices=[1]  OutputSizes=1
  Selector2 : Selector  InputPortWidth=2  IndexOptions=Index vector (dialog)  Indices=[1]  OutputSizes=1
  Selector3 : Selector  InputPortWidth=3  IndexOptions=Index vector (dialog)  Indices=[1]  OutputSizes=1
  Selector4 : Selector  InputPortWidth=2  IndexOptions=Index vector (dialog)  Indices=[1]  OutputSizes=1
  Selector5 : Selector  InputPortWidth=3  IndexOptions=Index vector (dialog)  Indices=[2]  OutputSizes=1
  Selector6 : Selector  InputPortWidth=2  IndexOptions=Index vector (dialog)  Indices=[2]  OutputSizes=1
  Selector7 : Selector  InputPortWidth=2  IndexOptions=Index vector (dialog)  Indices=[2]  OutputSizes=1
  Selector8 : Selector  InputPortWidth=2  IndexOptions=Index vector (dialog)  Indices=[2]  OutputSizes=1
  Terminator : Terminator
  Virtual Leg to Four Bar : MATLAB Function  TreatAsAtomicUnit=on
  Secondary Back/Front Motor Velocity [rad/s rad/s] : Outport
  Desired Swing Beta [rad rad/s rad/s^2] : Outport  Port=2
  wires:
  Demux4/1 -> Mux6/2
  Avoid Hitting Mechanical Limits/1(back_cmd) -> Mux3/1
  Avoid Hitting Mechanical Limits/4(dfront_cmd) -> Mux4/2
  Avoid Hitting Mechanical Limits/2(front_cmd) -> Mux3/2
  Avoid Hitting Mechanical Limits/5(ddback_cmd) -> Mux5/1
  Avoid Hitting Mechanical Limits/6(ddfront_cmd) -> Mux5/2
  Mux6/1 -> Back/Front PD/3(Measured Position [rad] [back front])
  Mux3/1 -> Back/Front PD/1(Desired Position [rad] [back front])
  Avoid Hitting Mechanical Limits/3(dback_cmd) -> Mux4/1
  Demux5/2 -> Mux11/1
  Secondary Front Gear [rad rad/s]/1 -> Demux4/1
  Mux4/1 -> Back/Front PD/2(Desired Velocity [rad/s] [back front])
  Z Desired [m m/s m/s^2]/1 -> "Convert COM Position to Joint Angles + Leg Length "/3(Z_star)
  Demux5/1 -> Mux6/1
  Secondary Back Gear [rad rad/s]/1 -> Demux5/1
  Demux6/4 -> Virtual Leg to Four Bar/4(phi)
  Virtual Leg to Four Bar/2(dback) -> Avoid Hitting Mechanical Limits/2(dback_desired)
  Mux11/1 -> Selector7/1, Selector1/1
  Virtual Leg to Four Bar/6(ddfront) -> Avoid Hitting Mechanical Limits/6(ddfront_desired)
  Virtual Leg to Four Bar/3(ddback) -> Avoid Hitting Mechanical Limits/3(ddback_desired)
  Demux6/6 -> Virtual Leg to Four Bar/6(ddphi)
  Virtual Leg to Four Bar/4(front) -> Avoid Hitting Mechanical Limits/4(front_desired)
  Demux6/5 -> Virtual Leg to Four Bar/5(dphi)
  Demux4/2 -> Mux11/2
  Virtual Leg to Four Bar/1(back) -> Avoid Hitting Mechanical Limits/1(back_desired)
  Torso Pitch [rad rad/s]/1 -> "Convert COM Position to Joint Angles + Leg Length "/8(pitch)
  Torso Roll [rad rad/s]/1 -> "Convert COM Position to Joint Angles + Leg Length "/7(roll)
  Right or Left Stance [1 or 0]/1 -> "Convert COM Position to Joint Angles + Leg Length "/4(right_left)
  Secondary Leg Roll [rad rad/s]/1 -> "Convert COM Position to Joint Angles + Leg Length "/10(lateral_angle)  "swing hip angle (lateral)"
  Secondary Leg Angle [rad rad/s]/1 -> "Convert COM Position to Joint Angles + Leg Length "/9(sagittal_angle)
  "Convert COM Position to Joint Angles + Leg Length "/2(desired_alpha) -> Mux8/2
  Secondary Leg Length [m m/s]/1 -> Selector6/1, Selector4/1, "Convert COM Position to Joint Angles + Leg Length "/11(leg_length)
  "Convert COM Position to Joint Angles + Leg Length "/1(desired_leg_length) -> Selector5/1, Selector3/1, Mux8/1
  Mux8/1 -> Demux6/1
  Y Desired [m m/s m/s^2]/1 -> "Convert COM Position to Joint Angles + Leg Length "/2(Y_star)
  Virtual Leg to Four Bar/5(dfront) -> Avoid Hitting Mechanical Limits/5(dfront_desired)
  Mux5/1 -> Terminator/1
  Pelvis to COM Position [m m m]/1 -> "Convert COM Position to Joint Angles + Leg Length "/5(com_pelvis_body)
  Pelvis to COM Velocity [m/s m/s m/s]/1 -> "Convert COM Position to Joint Angles + Leg Length "/6(dcom_pelvis_body)
  Mux12/1 -> Mirrored Back / Front Velocity Tracking/2
  Mux13/1 -> Mirrored Back / Front Velocity Tracking/1
  Selector1/1 -> Mux13/1
  Selector2/1 -> Mux13/2
  Selector7/1 -> Mux12/1
  Selector8/1 -> Mux12/2
  "Convert COM Position to Joint Angles + Leg Length "/3(desired_beta) -> Desired Swing Beta [rad rad/s rad/s^2]/1
  Back/Front PD/1(Commanded Velocity [rad/s] [back front]) -> Secondary Back/Front Motor Velocity [rad/s rad/s]/1, Selector8/1, Selector2/1
  X Desired [m m/s m/s^2]/1 -> "Convert COM Position to Joint Angles + Leg Length "/1(X_star)
  Mux1/1 -> Mirrored Leg Length Tracking/2
  Mux2/1 -> Mirrored Leg Length Tracking/1
  Selector3/1 -> Mux2/1
  Selector4/1 -> Mux2/2
  Selector5/1 -> Mux1/1
  Selector6/1 -> Mux1/2
  Avoid Virtual Leg Length Limits/1(l_leg_cmd) -> Virtual Leg to Four Bar/1(l_leg)
  Avoid Virtual Leg Length Limits/2(dl_leg_cmd) -> Virtual Leg to Four Bar/2(dl_leg)
  Avoid Virtual Leg Length Limits/3(ddl_leg_cmd) -> Virtual Leg to Four Bar/3(ddl_leg)
  Demux6/1 -> Avoid Virtual Leg Length Limits/1(l_leg_desired)
  Demux6/2 -> Avoid Virtual Leg Length Limits/2(dl_leg_desired)
  Demux6/3 -> Avoid Virtual Leg Length Limits/3(ddl_leg_desired)

== system deadbeat_running_control/Behavior/Compute Body Frame Accelerations ==
  accelerometer [g] x3 : Inport
  Convert to Body Frame IMU Accelerations : MATLAB Function  TreatAsAtomicUnit=on
  IMU Two Pole Filter2 : DiscreteTransferFcn  Numerator=[A_lpf_accelerometer 0 0]  Denominator=[1 B1_lpf_accelerometer B2_lpf_accelerometer]  InitialStates=[0, 0, g; 0, 0, g]*15.277  SampleTime=sample_time
  IMU XYZ Accelerations : Scope
  Mux : Mux  Inputs=2
  accelerations [m/s^2] x3 : Outport
  wires:
  accelerometer [g] x3/1 -> Convert to Body Frame IMU Accelerations/1(accelerometer)
  Convert to Body Frame IMU Accelerations/1(imu_accelerations) -> Mux/1, IMU Two Pole Filter2/1
  Mux/1 -> IMU XYZ Accelerations/1
  IMU Two Pole Filter2/1 -> Mux/2, accelerations [m/s^2] x3/1

== system deadbeat_running_control/Behavior/Compute Forces1 ==
  XYZ Acceleration : Inport
  Constant5 : Constant  Value=g
  Demux : Demux  Outputs=3
  Gain4 : Gain  Gain=m_total_real
  Mux : Mux  Inputs=3
  Sum8 : Sum  Inputs=|++
  XYZ Force : Outport
  wires:
  Constant5/1 -> Sum8/2
  XYZ Acceleration/1 -> Demux/1
  Gain4/1 -> XYZ Force/1
  Mux/1 -> Gain4/1
  Sum8/1 -> Mux/3
  Demux/3 -> Sum8/1
  Demux/2 -> Mux/2
  Demux/1 -> Mux/1

== system deadbeat_running_control/Behavior/Contact State Machine ==
  Contact Factor [body weight] : Inport
  "[Z dZ] [m m/s]" : Inport  Port=2
  Flight Time Remaining [s] : Inport  Port=3
  1-D Lookup Table : Lookup_n-D  NumberOfTableDimensions=1  BreakpointsForDimension1=[0.018, flight_duration]  Table=[contact_threshold, 1.0]  InternalRulePriority=Speed  RndMeth=Simplest  InputSameDT=on
  Contact Factor / Threshold : Scope
  Detect Fall Nonpositive : simulink/Logic and Bit Operations/Detect Fall Nonpositive  vinit=1  InputProcessing=Inherited  OutDataTypeStr=boolean
  Flight / Exiting Stance : Scope  NumInputPorts=2
  Logical Operator : Logic  Operator=NOT  AllPortsSameDT=off  OutDataTypeStr=boolean
  Mux : Mux  Inputs=2
  Mux25 : Mux
  Saturation : Saturate  UpperLimit=1.0  LowerLimit=contact_threshold
  Selector : Selector  InputPortWidth=2  IndexOptions=Index vector (dialog)  Indices=[2]  OutputSizes=1
  Stance On Or Off : Scope
  State Machine : State Transition Table  TreatAsAtomicUnit=on
  Terminator8 : Terminator
  Unit Delay5 : UnitDelay  SampleTime=-1
  Unit Delay6 : UnitDelay  SampleTime=sample_time
  Unit Delay7 : UnitDelay  InitialCondition=1  SampleTime=sample_time
  Unit Delay8 : UnitDelay  SampleTime=sample_time
  flight [1/0] : Outport
  Exiting Stance [1/0] : Outport  Port=2
  wires:
  "[Z dZ] [m m/s]"/1 -> Selector/1
  State Machine/1(" Touchdown") -> Mux25/1
  State Machine/2(" Unloading") -> Mux25/2
  Mux25/1 -> Unit Delay8/1
  State Machine/4(" Flight") -> Mux25/4, Unit Delay7/1
  Unit Delay5/1 -> State Machine/2(previous_z_velocity)
  Selector/1 -> Unit Delay5/1, State Machine/1(z_velocity)
  Unit Delay8/1 -> Terminator8/1
  State Machine/3(" Takeoff") -> Mux25/3, Unit Delay6/1
  Unit Delay6/1 -> Detect Fall Nonpositive/1
  Unit Delay7/1 -> Logical Operator/1, Flight / Exiting Stance/1, flight [1/0]/1
  Detect Fall Nonpositive/1 -> Flight / Exiting Stance/2, Exiting Stance [1/0]/1
  Flight Time Remaining [s]/1 -> 1-D Lookup Table/1
  1-D Lookup Table/1 -> Saturation/1
  Saturation/1 -> Mux/1, State Machine/4(variable_contact_threshold)
  Mux/1 -> Contact Factor / Threshold/1
  Contact Factor [body weight]/1 -> Mux/2, State Machine/3(contact_factor)
  Logical Operator/1 -> Stance On Or Off/1

== system deadbeat_running_control/Behavior/Desired Secondary Swing Targets ==
  Desired Primary X : Inport
  Desired Primary Z : Inport  Port=2
  Primary X,Y,Z : Inport  Port=3
  Primary dX,dY,dZ : Inport  Port=4
  Right / Left : Inport  Port=5
  Constant1 : Constant  Value=[lateral_target_position_right, 0]
  Constant2 : Constant  Value=[lateral_target_position_left, 0]
  Constant3 : Constant  Value=[z_retract_swing, 0]
  Constant4 : Constant  Value=0
  Constant5 : Constant  Value=0
  Constant6 : Constant  Value=0
  Demux{1..4} (4 alike) : Demux  Outputs=3
  Desired XYZ : Scope  NumInputPorts=4
  Fcn : Fcn  Expr=u - z_retract_swing
  Gain : Gain  Gain=-1
  Gain1 : Gain  Gain=-1
  Mux : Mux  Inputs=3
  Mux{25,29,32,34..35} (5 alike) : Mux  Inputs=2
  Primary Desired X and Z : Scope  NumInputPorts=2
  Primary XYZ : Scope  NumInputPorts=3
  Selector3 : Selector  InputPortWidth=3  IndexOptions=Index vector (dialog)  Indices=[1]  OutputSizes=1
  Selector4 : Selector  InputPortWidth=3  IndexOptions=Index vector (dialog)  Indices=[1]  OutputSizes=1
  Selector5 : Selector  InputPortWidth=3  IndexOptions=Index vector (dialog)  Indices=[1]  OutputSizes=1
  Sum2 : Sum  Inputs=-+|
  Switch1 : Switch  Criteria=u2 ~= 0
  Terminator : Terminator
  Terminator1 : Terminator
  Desired X : Outport
  Desired Y : Outport  Port=2
  Desired Z : Outport  Port=3
  wires:
  Demux2/2 -> Terminator/1
  Demux2/3 -> Mux35/2
  Demux1/3 -> Mux35/1
  Mux34/1 -> Gain/1
  Demux1/2 -> Terminator1/1
  Demux1/1 -> Mux34/1
  Demux2/1 -> Mux34/2
  Primary dX,dY,dZ/1 -> Demux2/1
  Primary X,Y,Z/1 -> Demux3/1, Demux1/1
  Gain/1 -> Mux32/1
  Constant6/1 -> Mux29/2
  Constant5/1 -> Mux25/2
  Constant4/1 -> Mux32/2
  Switch1/1 -> Mux25/1
  Right / Left/1 -> Desired XYZ/4, Switch1/2
  Constant1/1 -> Switch1/3
  Constant2/1 -> Switch1/1
  Sum2/1 -> Mux29/1
  Constant3/1 -> Sum2/1
  Mux35/1 -> Sum2/2
  Mux29/1 -> Selector5/1
  Mux25/1 -> Selector4/1, Desired Y/1
  Mux32/1 -> Selector3/1
  Selector3/1 -> Desired XYZ/1
  Selector5/1 -> Desired XYZ/3
  Selector4/1 -> Desired XYZ/2
  Demux3/1 -> Primary XYZ/1
  Demux3/2 -> Primary XYZ/2
  Demux3/3 -> Primary XYZ/3
  Gain1/1 -> Desired X/1
  Mux/1 -> Desired Z/1
  Desired Primary Z/1 -> Primary Desired X and Z/2, Demux4/1
  Demux4/3 -> Mux/3
  Demux4/2 -> Mux/2
  Demux4/1 -> Fcn/1
  Fcn/1 -> Mux/1
  Desired Primary X/1 -> Primary Desired X and Z/1, Gain1/1

== system deadbeat_running_control/Behavior/Estimate Angular Accelerations2 ==
  Angular Velocities [rad/s] x3 : Inport
  Enabled : Inport  Port=2
  Detect Change : simulink/Logic and Bit Operations/Detect Change  vinit=0  InputProcessing=Inherited  OutDataTypeStr=boolean
  Difference : simulink/Discrete/Difference  ICPrevInput=0.0  InputProcessing=Inherited  OutMin=[]  OutMax=[]  OutDataType=fixdt(1, 16)  OutScaling=2^-10  DoSatur=off
  Gain : Gain  Gain=1/sample_time
  IMU Two Pole Filter1 : DiscreteTransferFcn  Numerator=[A_lpf_imu 0 0]  Denominator=[1 B1_lpf_imu B2_lpf_imu]  SampleTime=sample_time
  Logical Operator5 : Logic  Operator=NOT  AllPortsSameDT=off  OutDataTypeStr=boolean
  Product : Product
  Angular Accelerations [rad/s^2] x3 : Outport
  wires:
  IMU Two Pole Filter1/1 -> Angular Accelerations [rad/s^2] x3/1
  Detect Change/1 -> Logical Operator5/1
  Difference/1 -> Gain/1
  Gain/1 -> Product/1
  Angular Velocities [rad/s] x3/1 -> Difference/1
  Product/1 -> IMU Two Pole Filter1/1
  Logical Operator5/1 -> Product/2
  Enabled/1 -> Detect Change/1

== system deadbeat_running_control/Behavior/Estimate Angular Accelerations3 ==
  Angular Velocities [rad/s] x2 : Inport
  Enabled : Inport  Port=2
  Detect Change : simulink/Logic and Bit Operations/Detect Change  vinit=0  InputProcessing=Inherited  OutDataTypeStr=boolean
  Difference : simulink/Discrete/Difference  ICPrevInput=0.0  InputProcessing=Inherited  OutMin=[]  OutMax=[]  OutDataType=fixdt(1, 16)  OutScaling=2^-10  DoSatur=off
  Gain : Gain  Gain=1/sample_time
  Lateral Angle Two Pole Filter1 : DiscreteTransferFcn  Numerator=[A_lpf_lateral_angle 0 0]  Denominator=[1 B1_lpf_lateral_angle B2_lpf_lateral_angle]  SampleTime=sample_time
  Logical Operator5 : Logic  Operator=NOT  AllPortsSameDT=off  OutDataTypeStr=boolean
  Product : Product
  Angular Accelerations [rad/s^2] x2 : Outport
  wires:
  Lateral Angle Two Pole Filter1/1 -> Angular Accelerations [rad/s^2] x2/1
  Enabled/1 -> Detect Change/1
  Logical Operator5/1 -> Product/2
  Product/1 -> Lateral Angle Two Pole Filter1/1
  Angular Velocities [rad/s] x2/1 -> Difference/1
  Gain/1 -> Product/1
  Difference/1 -> Gain/1
  Detect Change/1 -> Logical Operator5/1

== system deadbeat_running_control/Behavior/Exited Stance ==
  Enable : EnablePort  StatesWhenEnabling=reset
  Constant : Constant
  Takeoff? : Outport  InitialOutput=[0]
  wires:
  Constant/1 -> Takeoff?/1
